simulink model "comparacao_roda_adriane_estacio"  (R2016a)
settings: Solver=VariableStepAuto  StartTime=0.0  StopTime=100  RelTol=1e-3
InitFcn:
  | clear all;
  | Kpx = 10;
  | Kix = 25;
  | Kpy = 10;
  | Kiy = 25;
  | Kvphi = 3;
  | Kpphi = 2.25;
  | 
  | Kem = 0.0059;
  | Kti = 0.0059;
  | Vdi = 5.4;
  | R = 1.71;
  | r = 0.072;
  | eta = 0.83;
  | N = 19;
  | 
  | Jw = 8.1e-4;
  | 
  | mi = 0.25;
  | b = .1;
  | 
  | alpha1 = 0;
  | alpha2 = 120*pi/180;
  | alpha3 = 240*pi/180;
  | g = 9.8;
  | vs = 6e-10;
  | M = 1.83;
  | l1 = 0.09;
  | l2 = 0.09;
  | l3 = 0.09;
  | r1 = 0.072;
  | r2 = 0.072;
  | r3 = 0.072;
  | kt = 0.0059;
  | kem = 0.0059;
  | N = 19;
  | L = 0.00011;
  | R = 1.71;
  | Jm1 = 3.88e-7;
  | Jm2 = 3.88e-7;
  | Jm3 = 3.88e-7;
  | J1 = 8.1e-4;
  | J2 = 8.1e-4;
  | J3 = 8.1e-4;
  | J = 2.125;
  | eta = 0.83;
  | freq = 1000; % varia entre 2.5kHz e 5Mhz
  | mic = 0.46;
  | mis = 0.46;
  | sigma0 = 100;
  | sigma1 = 0.1;
  | sigma2 = 0.1;
  | 
  | mi = 0.25;
  | b = .1;
  | 
  | kctr = kt*5.4*eta*N/(R*r1)
settings Model: Creator=Pichau  LastModifiedBy=Pichau
settings DataIOCC: SignalLogging=off

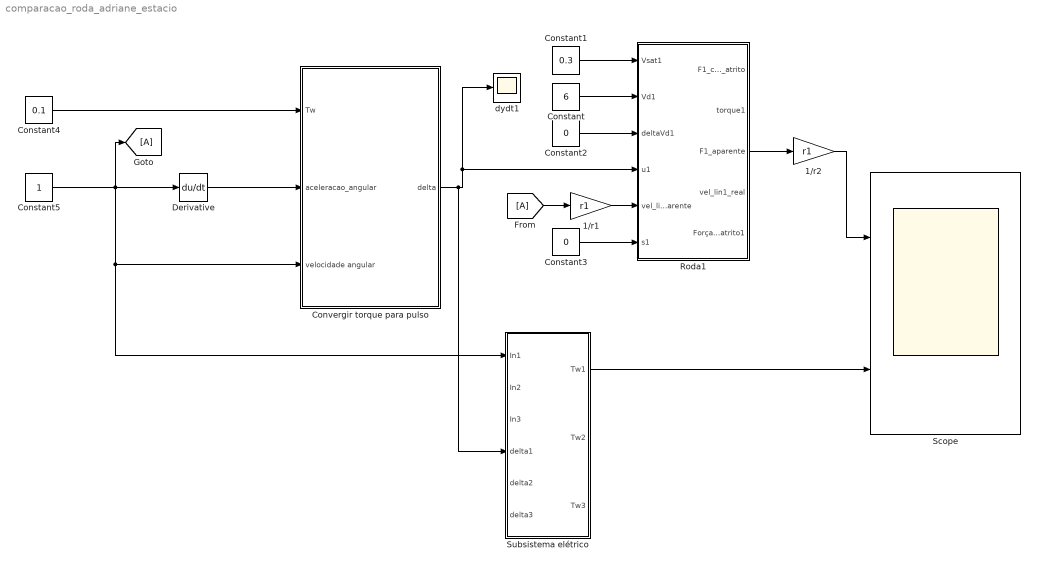
== system comparacao_roda_adriane_estacio ==
  1/r1 : Gain  Gain=r1
  1/r2 : Gain  Gain=r1
  Constant : Constant  Value=6
  Constant1 : Constant  Value=0.3
  Constant2 : Constant  Value=0
  Constant3 : Constant  Value=0
  Constant4 : Constant  Value=0.1
  Constant5 : Constant
  Convergir torque para pulso : Subsystem
  Derivative : Derivative
  Roda1 : Subsystem
  Scope : Scope  NumInputPorts=2
  Subsistema elétrico : Subsystem
  dydt1 : Scope
  wires:
  Convergir torque para pulso/1(delta) -> Subsistema elétrico/4(delta1), dydt1/1, Roda1/4(u1)
  Constant4/1 -> Convergir torque para pulso/1(Tw)
  Constant5/1 -> Derivative/1, [A], Subsistema elétrico/1(In1), Convergir torque para pulso/3(velocidade angular)
  Derivative/1 -> Convergir torque para pulso/2(aceleracao_angular)
  [A] -> 1/r1/1
  1/r1/1 -> Roda1/5(vel_lin1_aparente)
  Roda1/3(F1_aparente) -> 1/r2/1
  Constant/1 -> Roda1/2(Vd1)
  Constant1/1 -> Roda1/1(Vsat1)
  Constant2/1 -> Roda1/3(deltaVd1)
  Constant3/1 -> Roda1/6(s1)
  1/r2/1 -> Scope/1
  Subsistema elétrico/1(Tw1) -> Scope/2

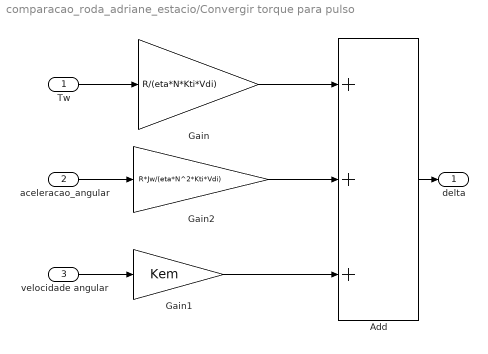
== system comparacao_roda_adriane_estacio/Convergir torque para pulso ==
  Tw : Inport
  aceleracao_angular : Inport  Port=2
  velocidade angular : Inport  Port=3
  Add : Sum  Inputs=+++
  Gain : Gain  Gain=R/(eta*N*Kti*Vdi)
  Gain1 : Gain  Gain=Kem
  Gain2 : Gain  Gain=R*Jw/(eta*N^2*Kti*Vdi)
  delta : Outport
  wires:
  aceleracao_angular/1 -> Gain2/1
  velocidade angular/1 -> Gain1/1
  Add/1 -> delta/1
  Tw/1 -> Gain/1
  Gain1/1 -> Add/3
  Gain/1 -> Add/1
  Gain2/1 -> Add/2

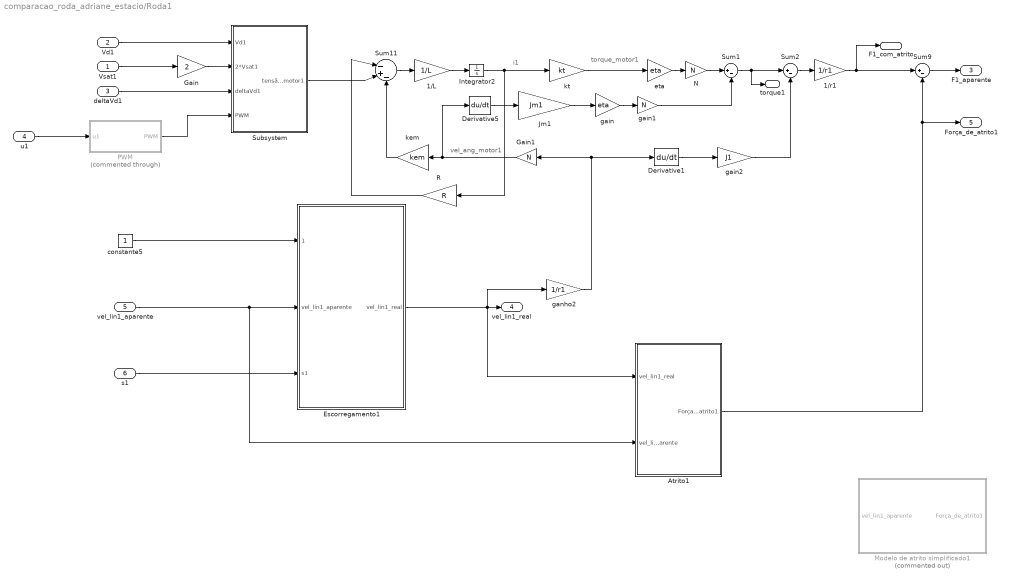
== system comparacao_roda_adriane_estacio/Roda1 ==
  note: i1
  note: torque_motor1
  note: vel_ang_motor1
  Vsat1 : Inport
  Vd1 : Inport  Port=2
  deltaVd1 : Inport  Port=3
  u1 : Inport  Port=4
  vel_lin1_aparente : Inport  Port=5
  s1 : Inport  Port=6
  1/L : Gain  Gain=1/L
  1/r1 : Gain  Gain=1/r1
  Atrito1 : Subsystem
  Derivative1 : Derivative
  Derivative5 : Derivative
  Escorregamento1 : Subsystem
  Gain : Gain  Gain=2
  Gain1 : Gain  Gain=N
  Integrator2 : Integrator
  Jm1 : Gain  Gain=Jm1
  Modelo de atrito simplificado1 : Subsystem  Commented=on
  N : Gain  Gain=N
  PWM : Subsystem  Commented=through
  R : Gain  Gain=R
  Subsystem : Subsystem
  Sum1 : Sum  Inputs=|+-
  Sum11 : Sum  Inputs=|-+-
  Sum2 : Sum  Inputs=|+-
  Sum9 : Sum  Inputs=|+-
  constante5 : Constant
  eta : Gain  Gain=eta
  gain : Gain  Gain=eta
  gain1 : Gain  Gain=N
  gain2 : Gain  Gain=J1
  ganho2 : Gain  Gain=1/r1
  kem : Gain  Gain=kem
  kt : Gain  Gain=kt
  F1_com_atrito : Outport
  torque1 : Outport  Port=2
  F1_aparente : Outport  Port=3
  vel_lin1_real : Outport  Port=4
  Força_de_atrito1 : Outport  Port=5
  wires:
  Derivative5/1 -> Jm1/1
  Sum11/1 -> 1/L/1
  1/L/1 -> Integrator2/1
  Integrator2/1 -> kt/1, R/1
  Subsystem/1(tensão_motor1) -> Sum11/2
  kt/1 -> eta/1
  eta/1 -> N/1
  Gain1/1 -> kem/1, Derivative5/1
  1/r1/1 -> Sum9/1, F1_com_atrito/1
  Vsat1/1 -> Gain/1
  Vd1/1 -> Subsystem/1(Vd1)
  deltaVd1/1 -> Subsystem/3(deltaVd1)
  Gain/1 -> Subsystem/2("2*Vsat1 ")
  N/1 -> Sum1/1
  Sum1/1 -> torque1/1, Sum2/1
  gain/1 -> gain1/1
  Jm1/1 -> gain/1
  gain1/1 -> Sum1/2
  Derivative1/1 -> gain2/1
  gain2/1 -> Sum2/2
  Sum2/1 -> 1/r1/1
  kem/1 -> Sum11/3
  R/1 -> Sum11/1
  Sum9/1 -> F1_aparente/1
  u1/1 -> PWM/1(u1)
  Escorregamento1/1("vel_lin1_real ") -> Atrito1/1(vel_lin1_real), ganho2/1, vel_lin1_real/1
  ganho2/1 -> Derivative1/1, Gain1/1
  Atrito1/1(Força_de_atrito1) -> Sum9/2, Força_de_atrito1/1
  constante5/1 -> Escorregamento1/1(1)
  s1/1 -> Escorregamento1/3(s1)
  vel_lin1_aparente/1 -> Atrito1/2("vel_lin1_aparente "), Escorregamento1/2("vel_lin1_aparente ")
  PWM/1(PWM) -> Subsystem/4(PWM)

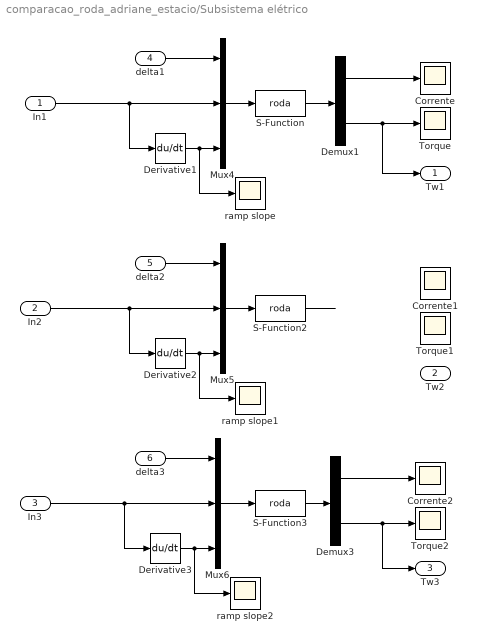
== system comparacao_roda_adriane_estacio/Subsistema elétrico ==
  In1 : Inport
  In2 : Inport  Port=2
  In3 : Inport  Port=3
  delta1 : Inport  Port=4
  delta2 : Inport  Port=5
  delta3 : Inport  Port=6
  Corrente : Scope
  Corrente1 : Scope
  Corrente2 : Scope
  Demux1 : Demux  Outputs=2
  Demux3 : Demux  Outputs=2
  Derivative1 : Derivative
  Derivative2 : Derivative
  Derivative3 : Derivative
  Mux4 : Mux  Inputs=3
  Mux5 : Mux  Inputs=3
  Mux6 : Mux  Inputs=3
  S-Function : S-Function  FunctionName=roda  Parameters=Vd,Vsat,deltaVd,L,Kem,R,Kti,Jm,eta,N  SFunctionDeploymentMode=off  EnableBusSupport=off  mask{Vd=6, Vsat=0.3, deltaVd=0, L=0.00011, Kem=0.0059, R=1.71, Kti=0.0059, Jm=3.88e-7, eta=0.83, N=19}
  S-Function2 : S-Function  FunctionName=roda  Parameters=Vd,Vsat,deltaVd,L,Kem,R,Kti,Jm,eta,N  SFunctionDeploymentMode=off  EnableBusSupport=off  mask{Vd=6, Vsat=0.3, deltaVd=0, L=0.00011, Kem=0.0059, R=1.71, Kti=0.0059, Jm=3.88e-7, eta=0.83, N=19}
  S-Function3 : S-Function  FunctionName=roda  Parameters=Vd,Vsat,deltaVd,L,Kem,R,Kti,Jm,eta,N  SFunctionDeploymentMode=off  EnableBusSupport=off  mask{Vd=6, Vsat=0.3, deltaVd=0, L=0.00011, Kem=0.0059, R=1.71, Kti=0.0059, Jm=3.88e-7, eta=0.83, N=19}
  Torque : Scope
  Torque1 : Scope
  Torque2 : Scope
  ramp slope : Scope
  ramp slope1 : Scope
  ramp slope2 : Scope
  Tw1 : Outport
  Tw2 : Outport  Port=2
  Tw3 : Outport  Port=3
  wires:
  Demux3/1 -> Corrente2/1
  Mux6/1 -> S-Function3/1
  Derivative3/1 -> ramp slope2/1, Mux6/3
  Demux3/2 -> Tw3/1, Torque2/1
  In3/1 -> Mux6/2, Derivative3/1
  S-Function3/1 -> Demux3/1
  delta2/1 -> Mux5/1
  delta3/1 -> Mux6/1
  Mux5/1 -> S-Function2/1
  In2/1 -> Derivative2/1, Mux5/2
  S-Function2/1 -> ?
  ? -> Corrente1/1
  ? -> Tw2/1, Torque1/1
  Derivative2/1 -> Mux5/3, ramp slope1/1
  Derivative1/1 -> ramp slope/1, Mux4/3
  In1/1 -> Mux4/2, Derivative1/1
  Demux1/2 -> Tw1/1, Torque/1
  Mux4/1 -> S-Function/1
  S-Function/1 -> Demux1/1
  delta1/1 -> Mux4/1
  Demux1/1 -> Corrente/1

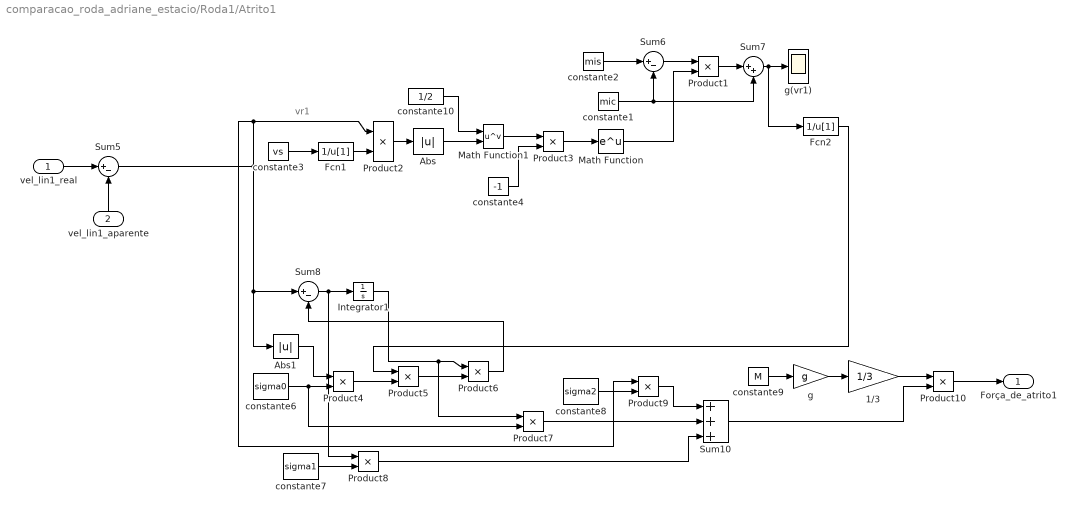
== system comparacao_roda_adriane_estacio/Roda1/Atrito1 ==
  note: vr1
  vel_lin1_real : Inport
  "vel_lin1_aparente " : Inport  Port=2
  1/3 : Gain  Gain=1/3
  Abs : Abs
  Abs1 : Abs
  Fcn1 : Fcn  Expr=1/u[1]
  Fcn2 : Fcn  Expr=1/u[1]
  Integrator1 : Integrator
  Math Function : Math  SaturateOnIntegerOverflow=on
  Math Function1 : Math  Operator=pow  SaturateOnIntegerOverflow=on
  Product{1..10} (10 alike) : Product  RndMeth=Zero
  Sum10 : Sum  Inputs=+++
  Sum5 : Sum  Inputs=|+-
  Sum6 : Sum  Inputs=|+-
  Sum7 : Sum  Inputs=|++
  Sum8 : Sum  Inputs=|+-
  constante1 : Constant  Value=mic
  constante10 : Constant  Value=1/2
  constante2 : Constant  Value=mis
  constante3 : Constant  Value=vs
  constante4 : Constant  Value=-1
  constante6 : Constant  Value=sigma0
  constante7 : Constant  Value=sigma1
  constante8 : Constant  Value=sigma2
  constante9 : Constant  Value=M
  g : Gain  Gain=g
  g(vr1) : Scope
  Força_de_atrito1 : Outport
  wires:
  constante2/1 -> Sum6/1
  constante1/1 -> Sum6/2, Sum7/2
  Sum6/1 -> Product1/1
  constante3/1 -> Fcn1/1
  Fcn1/1 -> Product2/2
  Sum5/1 -> Sum8/1, Abs1/1, Product9/1, Product2/1
  Product2/1 -> Abs/1
  Abs/1 -> Math Function1/2
  Math Function1/1 -> Product3/1
  constante4/1 -> Product3/2
  Product3/1 -> Math Function/1
  Math Function/1 -> Product1/2
  Product1/1 -> Sum7/1
  Sum7/1 -> g(vr1)/1, Fcn2/1
  Sum8/1 -> Integrator1/1, Product8/1
  Integrator1/1 -> Product6/1, Product7/1
  constante6/1 -> Product4/2, Product7/2
  Abs1/1 -> Product4/1
  Product4/1 -> Product5/2
  Fcn2/1 -> Product5/1
  Product5/1 -> Product6/2
  Product6/1 -> Sum8/2
  constante7/1 -> Product8/2
  Product8/1 -> Sum10/3
  Product7/1 -> Sum10/2
  constante8/1 -> Product9/2
  Product9/1 -> Sum10/1
  constante9/1 -> g/1
  g/1 -> 1/3/1
  1/3/1 -> Product10/1
  Sum10/1 -> Product10/2
  constante10/1 -> Math Function1/1
  vel_lin1_real/1 -> Sum5/1
  "vel_lin1_aparente "/1 -> Sum5/2
  Product10/1 -> Força_de_atrito1/1

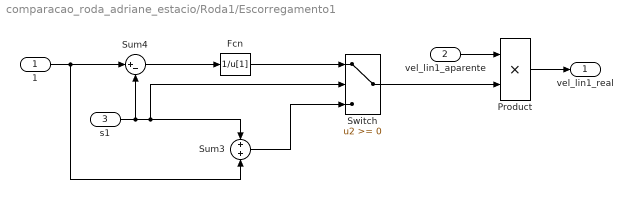
== system comparacao_roda_adriane_estacio/Roda1/Escorregamento1 ==
  1 : Inport
  "vel_lin1_aparente " : Inport  Port=2
  s1 : Inport  Port=3
  Fcn : Fcn  Expr=1/u[1]
  Product : Product  RndMeth=Zero
  Sum3 : Sum  Inputs=+|+
  Sum4 : Sum  Inputs=|+-
  Switch : Switch
  "vel_lin1_real " : Outport
  wires:
  s1/1 -> Switch/2, Sum3/1, Sum4/2
  1/1 -> Sum3/2, Sum4/1
  Sum4/1 -> Fcn/1
  Fcn/1 -> Switch/1
  Sum3/1 -> Switch/3
  Switch/1 -> Product/2
  "vel_lin1_aparente "/1 -> Product/1
  Product/1 -> "vel_lin1_real "/1

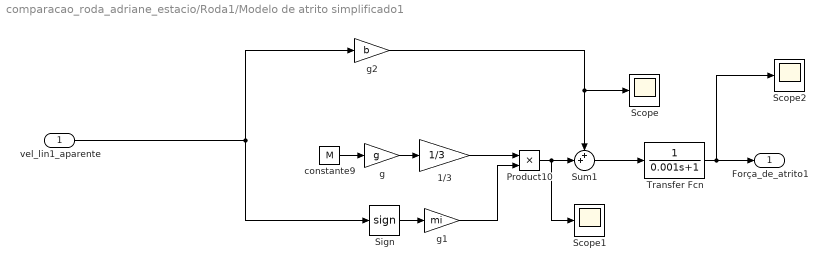
== system comparacao_roda_adriane_estacio/Roda1/Modelo de atrito simplificado1 ==
  vel_lin1_aparente : Inport
  1/3 : Gain  Gain=1/3
  Product10 : Product  RndMeth=Zero
  Scope : Scope
  Scope1 : Scope
  Scope2 : Scope
  Sign : Signum
  Sum1 : Sum  Inputs=++|
  Transfer Fcn : TransferFcn  Denominator=[0.001 1]
  constante9 : Constant  Value=M
  g : Gain  Gain=g
  g1 : Gain  Gain=mi
  g2 : Gain  Gain=b
  Força_de_atrito1 : Outport
  wires:
  Transfer Fcn/1 -> Força_de_atrito1/1, Scope2/1
  g2/1 -> Scope/1, Sum1/1
  Sum1/1 -> Transfer Fcn/1
  Sign/1 -> g1/1
  vel_lin1_aparente/1 -> Sign/1, g2/1
  Product10/1 -> Sum1/2, Scope1/1
  g1/1 -> Product10/2
  1/3/1 -> Product10/1
  g/1 -> 1/3/1
  constante9/1 -> g/1

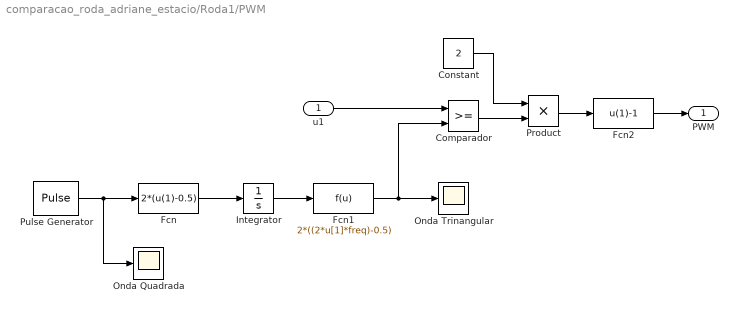
== system comparacao_roda_adriane_estacio/Roda1/PWM ==
  u1 : Inport
  Comparador : RelationalOperator  OutDataTypeStr=boolean
  Constant : Constant  Value=2
  Fcn : Fcn  Expr=2*(u(1)-0.5)
  Fcn1 : Fcn  Expr=2*((2*u[1]*freq)-0.5)
  Fcn2 : Fcn  Expr=u(1)-1
  Integrator : Integrator
  Onda Quadrada : Scope
  Onda Trinangular : Scope
  Product : Product  RndMeth=Zero
  Pulse Generator : DiscretePulseGenerator  PulseType=Time based  Period=1/freq  PulseWidth=50
  PWM : Outport
  wires:
  Pulse Generator/1 -> Fcn/1, Onda Quadrada/1
  Fcn/1 -> Integrator/1
  Integrator/1 -> Fcn1/1
  Fcn1/1 -> Onda Trinangular/1, Comparador/2
  u1/1 -> Comparador/1
  Fcn2/1 -> PWM/1
  Comparador/1 -> Product/2
  Product/1 -> Fcn2/1
  Constant/1 -> Product/1

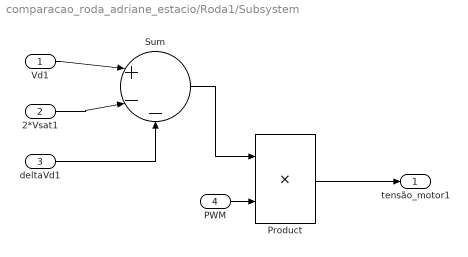
== system comparacao_roda_adriane_estacio/Roda1/Subsystem ==
  Vd1 : Inport
  "2*Vsat1 " : Inport  Port=2
  deltaVd1 : Inport  Port=3
  PWM : Inport  Port=4
  Product : Product  RndMeth=Zero
  Sum : Sum  Inputs=|+--
  tensão_motor1 : Outport
  wires:
  Sum/1 -> Product/1
  Vd1/1 -> Sum/1
  Product/1 -> tensão_motor1/1
  PWM/1 -> Product/2
  deltaVd1/1 -> Sum/3
  "2*Vsat1 "/1 -> Sum/2
